simulink model "sim_tanque"  (Simulink 8.3)
settings: Solver=ode15s  StartTime=0.0  StopTime=20  RelTol=1e-3
InitFcn:
  | matrizes_jacob
values from neighbouring files (symbols this model uses):
  A = sym(zeros(1,N+1))    [gainSchedule_Pade_2.m]    (also in matrizes_jacob.m = double(subs(jacobian(f,x))); pade_symbolic_gainSchedule_1.m = sym('A', [1 N+1]); test_Pade.m = sym('A', [1 N+1]))
  B = (Cmat \ rhs).'    [gainSchedule_Pade_2.m]    (also in matrizes_jacob.m = double(subs(jacobian(f,u))); pade_symbolic_gainSchedule_1.m = sym('B', [1 M]); test_Pade.m = sym('B', [1 M]))
  C = eye(2)    [matrizes_jacob.m]
  D = zeros(2,3)    [matrizes_jacob.m]
settings Model: Creator=marcio  LastModifiedBy=marcio
settings OptimizationCC: ExpressionDepthLimit=2147483647
settings DebuggingCC: SolverPrmCheckMsg=none  FcnCallInpInsideContextMsg=UseLocalSettings

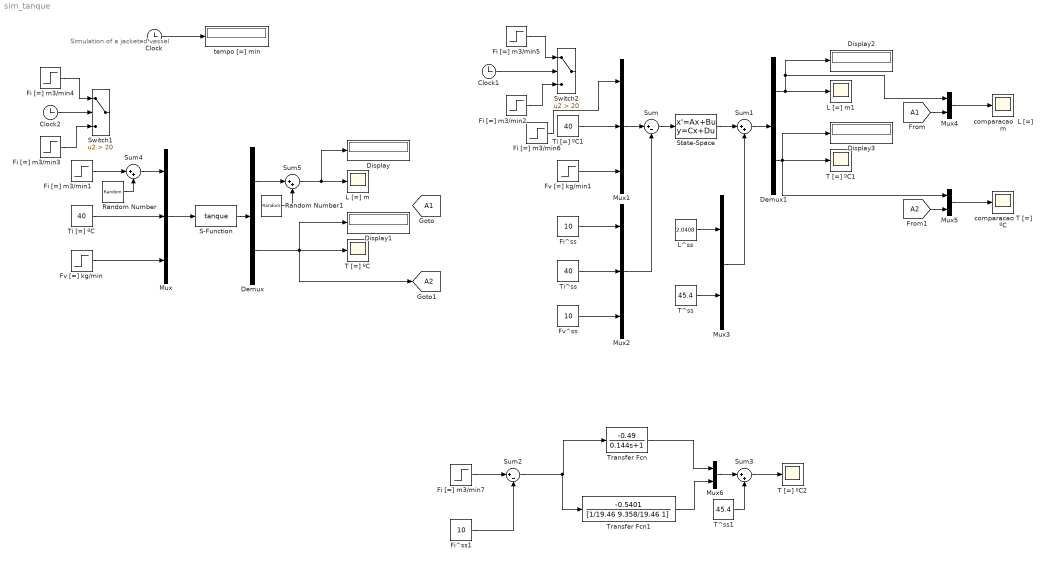
== system sim_tanque ==
  note: Simulation of a jacketed vessel
  Clock : Clock
  Clock1 : Clock
  Clock2 : Clock
  Demux : Demux  Outputs=2
  Demux1 : Demux  Outputs=2
  Display{,1..3} (4 alike) : Display
  Fi [=] m3/min1 : Step  Time=2  Before=10  After=11  SampleTime=0
  Fi [=] m3/min2 : Step  Time=2  Before=10  After=15  SampleTime=0
  Fi [=] m3/min3 : Step  Time=2  Before=10  After=14  SampleTime=0
  Fi [=] m3/min4 : Step  Time=10  Before=14  After=10  SampleTime=0
  Fi [=] m3/min5 : Step  Time=10  Before=15  After=10  SampleTime=0
  Fi [=] m3/min6 : Step  Time=2  Before=10  After=11  SampleTime=0
  Fi [=] m3/min7 : Step  Time=2  Before=10  After=11  SampleTime=0
  Fi^ss : Constant  Value=10
  Fi^ss1 : Constant  Value=10
  Fv [=] kg/min : Step  Time=20  Before=10  After=10  SampleTime=0
  Fv [=] kg/min1 : Step  Time=20  Before=10  After=10  SampleTime=0
  Fv^ss : Constant  Value=10
  L [=] m : Scope
  L [=] m1 : Scope
      settings: SaveName=ScopeData2
  L^ss : Constant  Value=2.0408
  Mux : Mux  Inputs=3
  Mux1 : Mux  Inputs=3
  Mux2 : Mux  Inputs=3
  Mux{3..6} (4 alike) : Mux  Inputs=2
  Random Number : RandomNumber  Variance=0.1  SampleTime=0.1
  Random Number1 : RandomNumber  Variance=0.001  SampleTime=0.1
  S-Function : S-Function  FunctionName=tanque  Parameters=rho,Cp,At,k,lambda  EnableBusSupport=off  mask{rho=1e3, Cp=4.18, At=pi*0.5^2, k=7, lambda=2.257e4}
      mask prompts: rho "massa especifica [=] kg/m3"; Cp "calor especifico [=] kJ/kg.ºC"; At "area transversal [=] m2"; k "constante da valvula [=] m^2.5/min"; lambda "calor de vaporizacao [=] kJ/kg"
  State-Space : StateSpace  A=A  B=B  C=C  D=D  X0=[0 0]
  Sum : Sum  Inputs=|+-
  Sum{1,3..5} (4 alike) : Sum  Inputs=|++
  Sum2 : Sum  Inputs=|+-
  Switch1 : Switch  Criteria=u2 > Threshold  Threshold=20
  Switch2 : Switch  Criteria=u2 > Threshold  Threshold=20
  T [=] ºC : Scope
  T [=] ºC1 : Scope
      settings: SaveName=ScopeData3
  T [=] ºC2 : Scope
      settings: SaveName=ScopeData6
  T^ss : Constant  Value=45.4
  T^ss1 : Constant  Value=45.4
  Ti [=] ºC : Constant  Value=40
  Ti [=] ºC1 : Constant  Value=40
  Ti^ss : Constant  Value=40
  Transfer Fcn : TransferFcn  Numerator=[-0.49]  Denominator=[0.144 1]
  Transfer Fcn1 : TransferFcn  Numerator=[-0.5401]  Denominator=[1/19.46 9.358/19.46 1]
  comparacao T [=] ºC : Scope
      settings: SaveName=ScopeData5
  comparacao  L [=] m : Scope
      settings: SaveName=ScopeData4
  tempo [=] min : Display
  tag scope: A1=global, A2=global
  wires:
  Mux/1 -> S-Function/1
  S-Function/1 -> Demux/1
  Demux/2 -> [A2], T [=] ºC/1, Display1/1
  Ti [=] ºC/1 -> Mux/2
  Fv [=] kg/min/1 -> Mux/3
  Clock/1 -> tempo [=] min/1
  Ti [=] ºC1/1 -> Mux1/2
  Fv [=] kg/min1/1 -> Mux1/3
  Demux1/1 -> Mux4/1, Display2/1, L [=] m1/1
  Demux1/2 -> Mux5/1, Display3/1, T [=] ºC1/1
  Fi^ss/1 -> Mux2/1
  Ti^ss/1 -> Mux2/2
  Fv^ss/1 -> Mux2/3
  Mux1/1 -> Sum/1
  Mux2/1 -> Sum/2
  Sum/1 -> State-Space/1
  State-Space/1 -> Sum1/1
  Sum1/1 -> Demux1/1
  Mux3/1 -> Sum1/2
  L^ss/1 -> Mux3/1
  T^ss/1 -> Mux3/2
  [A1] -> Mux4/2
  Mux4/1 -> comparacao  L [=] m/1
  [A2] -> Mux5/2
  Mux5/1 -> comparacao T [=] ºC/1
  Clock2/1 -> Switch1/2
  Fi [=] m3/min4/1 -> Switch1/1
  Fi [=] m3/min3/1 -> Switch1/3
  Clock1/1 -> Switch2/2
  Fi [=] m3/min5/1 -> Switch2/1
  Fi [=] m3/min2/1 -> Switch2/3
  Fi [=] m3/min6/1 -> Mux1/1
  Transfer Fcn/1 -> Mux6/1
  Transfer Fcn1/1 -> Mux6/2
  Fi [=] m3/min7/1 -> Sum2/1
  Fi^ss1/1 -> Sum2/2
  Sum2/1 -> Transfer Fcn1/1, Transfer Fcn/1
  Mux6/1 -> Sum3/1
  T^ss1/1 -> Sum3/2
  Sum3/1 -> T [=] ºC2/1
  Fi [=] m3/min1/1 -> Sum4/1
  Random Number/1 -> Sum4/2
  Sum4/1 -> Mux/1
  Demux/1 -> Sum5/1
  Random Number1/1 -> Sum5/2
  Sum5/1 -> Display/1, L [=] m/1
